simulink model "Fig1"  (R2023b)
settings: Solver=VariableStepAuto  StartTime=0.0  StopTime=simTime  RelTol=1e-3
values from neighbouring files (symbols this model uses):
  deltaT = 15    [Bird.m]    (also in BirdNoSim.m = 10)
  I = 2119    [Bird.m]    (also in BirdNoSim.m; DelaySweep.mat; NoiseSweep.mat; bird__pd_control.m = 0.002119)
  Ki = K    (= 9)    [Bird.m]
  Kp = K*tauC    (= 360)    [Bird.m]
  tauP = 69.7    [Bird.m]    (also in BirdNoSim.m = 0.0697)
settings Model: Creator=haydenwalker  LastModifiedBy=haydenwalker
settings DataIOCC: SaveFormat=Array

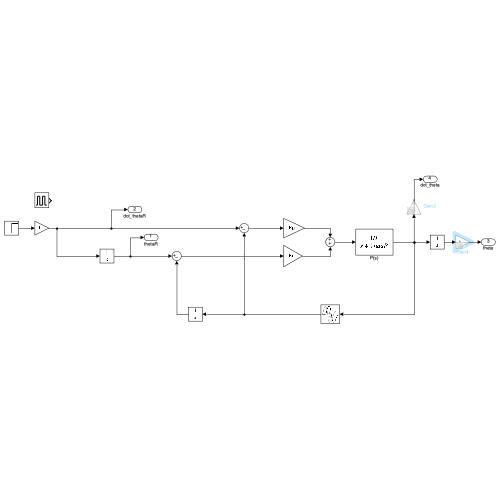
[thumbnail: Simulink's stored preview of the top-level diagram]
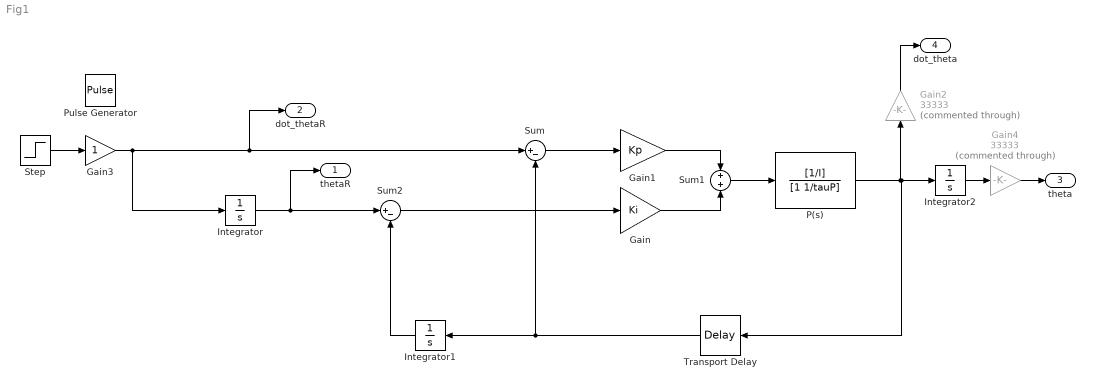
== system Fig1 ==
  Gain : Gain  Gain=Ki
  Gain1 : Gain  Gain=Kp
  Gain2 : Gain  Commented=through  Gain=33333
  Gain3 : Gain
  Gain4 : Gain  Commented=through  Gain=33333
  Integrator : Integrator
  Integrator1 : Integrator
  Integrator2 : Integrator
  P(s) : TransferFcn  Numerator=[1/I]  Denominator=[1 1/tauP]
  Pulse Generator : DiscretePulseGenerator  PulseType=Time based  Period=10  PulseWidth=10
  Step : Step  SampleTime=0
  Sum : Sum  Inputs=|+-
  Sum1 : Sum  Inputs=+|+
  Sum2 : Sum  Inputs=|+-
  Transport Delay : TransportDelay  DelayTime=deltaT
  thetaR : Outport  OutDataTypeStr=double
  dot_thetaR : Outport  Port=2  OutDataTypeStr=double
  theta : Outport  Port=3  OutDataTypeStr=double
  dot_theta : Outport  Port=4  OutDataTypeStr=double
  wires:
  Gain1/1 -> Sum1/1
  Gain/1 -> Sum1/2
  Sum1/1 -> P(s)/1
  P(s)/1 -> Transport Delay/1, Integrator2/1, Gain2/1
  Integrator1/1 -> Sum2/2
  Sum2/1 -> Gain/1
  Sum/1 -> Gain1/1
  Transport Delay/1 -> Sum/2, Integrator1/1
  Integrator2/1 -> Gain4/1
  Integrator/1 -> thetaR/1, Sum2/1
  Gain3/1 -> Integrator/1, dot_thetaR/1, Sum/1
  Step/1 -> Gain3/1
  Gain2/1 -> dot_theta/1
  Gain4/1 -> theta/1
